simulink model "SlidingMode_hysteresis"  (R2024a)
settings: Solver=ode45  StartTime=0.0  StopTime=Tsim  RelTol=1e-3  EnableMultiTasking=on
undefined symbols (not defined in the file): delta, xInit
settings Model: Creator=DRijlaars  LastModifiedBy=bengo
settings SolverCC: AlgebraicLoopSolver=TrustRegion
settings DataIOCC: LimitDataPoints=on  SaveFormat=Array  SignalLoggingSaveFormat=ModelDataLogs  ReturnWorkspaceOutputs=off
settings OptimizationCC: ExpressionDepthLimit=2147483647  InitFltsAndDblsToZero=on  LifeSpan=inf
settings DebuggingCC: UnderspecifiedInitializationDetection=Classic  MergeDetectMultiDrivingBlocksExec=none  SolverPrmCheckMsg=warning  FcnCallInpInsideContextMsg=warning  UnconnectedInputMsg=warning  UnconnectedOutputMsg=warning  UnconnectedLineMsg=warning  StateNameClashWarn=warning  SFUnexpectedBacktrackingDiag=warning  SFNoUnconditionalDefaultTransitionDiag=warning  SFExecutionAtInitializationDiag=none  ArithmeticOperatorsInVariantConditions=warning
settings HardwareCC: ProdBitPerPointer=32  ProdBitPerSizeT=32  ProdBitPerPtrDiffT=32  ProdLargestAtomicFloat=None  ProdIntDivRoundTo=Undefined  ProdEndianess=Unspecified  ProdWordSize=32  ProdHWDeviceType=32-bit Generic
settings ModelReferenceCC: PropagateSignalLabelsOutOfModel=off
settings SFSimCC: SimUseLocalCustomCode=off  CustomCodeUndefinedFunction=UseInterfaceOnly
settings RTWCC: RTWUseLocalCustomCode=off  GPUComputeCapability=3.5
settings CodeAppCC: StateflowObjectComments=on
settings GRTTargetCC: TargetLangStandard=C89/C90 (ANSI)  CombineOutputUpdateFcns=off  GRTInterface=on
settings ConfigComp: CovMetricSettings=dw  CovSaveCumulativeToWorkspaceVar=on  CovSaveSingleToWorkspaceVar=on  CovExternalEMLEnable=off

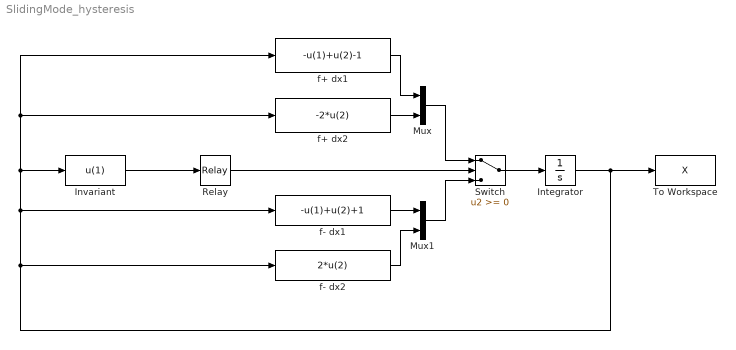
== system SlidingMode_hysteresis ==
  Integrator : Integrator  InitialCondition=xInit
  Invariant : Fcn  Expr=u(1)
  Mux : Mux  Inputs=2
  Mux1 : Mux  Inputs=2
  Relay : Relay  OnSwitchValue=delta  OffSwitchValue=-delta  OnOutputValue=0.01  OffOutputValue=-0.01
  Switch : Switch  SaturateOnIntegerOverflow=off  InputSameDT=off
  To Workspace : ToWorkspace  VariableName=X  SaveFormat=Timeseries  SampleTime=-1
  f+ dx1 : Fcn  Expr=-u(1)+u(2)-1
  f+ dx2 : Fcn  Expr=-2*u(2)
  f- dx1 : Fcn  Expr=-u(1)+u(2)+1
  f- dx2 : Fcn  Expr=2*u(2)
  wires:
  Integrator/1 -> To Workspace/1, f- dx2/1, Invariant/1, f+ dx1/1, f+ dx2/1, f- dx1/1
  Switch/1 -> Integrator/1
  Invariant/1 -> Relay/1
  Mux/1 -> Switch/1
  Mux1/1 -> Switch/3
  f- dx1/1 -> Mux1/1
  f- dx2/1 -> Mux1/2
  f+ dx2/1 -> Mux/2
  f+ dx1/1 -> Mux/1
  Relay/1 -> Switch/2
